simulink library "ModG_Vehiculo"  (R2018a)
settings: Solver=VariableStepAuto  StartTime=0.0  StopTime=10.0  RelTol=1e-3
undefined symbols (not defined in the file): a1, a2, Auto, b1d, b1i, b2d, b2i, b_sus, g, h, Iyy, Izz, Jw, k_sus, L, m, Rg, T1, T2
libraries: $bdroot x12, ModG_Neumatico x10, ModG_Transformaciones x2
settings Model: Creator=Lisandro Cocca  LastModifiedBy=Lisandro Cocca

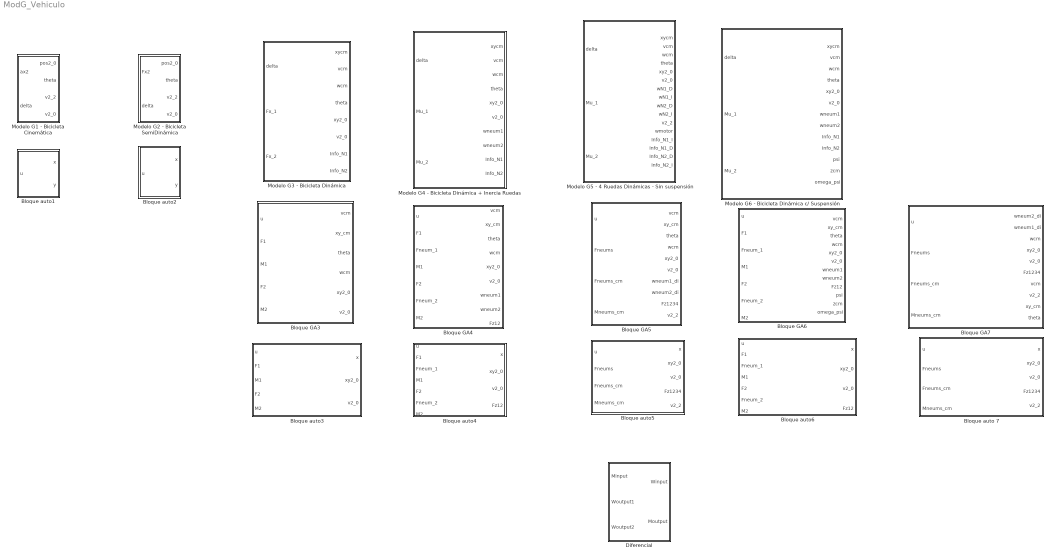
== system ModG_Vehiculo ==
  Bloque GA3 : Subsystem
  Bloque GA4 : Subsystem
  Bloque GA5 : Subsystem
  Bloque GA6 : Subsystem
  Bloque GA7 : Subsystem
  "Bloque auto 7 " : Subsystem
  Bloque auto1 : Subsystem
  Bloque auto2 : Subsystem
  Bloque auto3 : Subsystem
  Bloque auto4 : Subsystem
  Bloque auto5 : Subsystem
  Bloque auto6 : Subsystem
  Diferencial : Subsystem  mask{rel_dif=1}
      mask prompts: rel_dif "Relacion del diferencial 'rel_dif'"
  Modelo G1 - Bicicleta Cinemática : Subsystem  mask{L=L}
      mask prompts: L "Largo del auto "L" [m]"
  Modelo G2 - Bicicleta SemiDinámica : Subsystem  mask{L=L, m=m}
      mask prompts: L "Largo del auto "L" [m]"; m "Masa del auto "m" [kg]"
  Modelo G3 - Bicicleta Dinámica : Subsystem  mask{m=0, Izz=0, L=0, a2=0, a1=0, g=9.81}
      mask prompts: m "Masa del auto 'm' [kg]"; Izz "Momento de inercia respecto eje Z 'Izz' [kg/m^2]"; L "Distancia entre ejes 'L' [m]"; a2 "Distancia CM-Eje trasero 'a2' [m] (Numero positivo)"; a1 "Distancia CM-Eje delantero 'a1' [m] (Numero positivo)"; g "Aceleracion de la gravedad 'g' [m/s^2]"
  Modelo G4 - Bicicleta Dinámica + Inercia Ruedas : Subsystem  mask{m=0, Izz=0, L=0, a2=0, a1=0, h=0, g=9.81, GR=0, Rg=0, Jw=0}
      mask prompts: m "Masa del auto 'm' [kg]"; Izz "Momento de inercia respecto eje Z 'Izz' [kg/m^2]"; L "Distancia entre ejes 'L' [m]"; a2 "Distancia CM-Eje trasero 'a2' [m] (Numero positivo)"; a1 "Distancia CM-Eje delantero 'a1' [m] (Numero positivo)"; h "Altura del centro de masa 'h' [m]"; g "Aceleracion de la gravedad 'g' [m/s^2]"; GR "Gear Ratio 'GR'"; Rg "Radio Neumático 'Rg'"; Jw "Inercia Neumático 'Jw'"
  Modelo G5 - 4 Ruedas Dinámicas - Sin suspensión : Subsystem  mask{m=0, Izz=0, L=0, a2=0, a1=0, T1=0, b1d=0, b1i=0, b2d=0, b2i=0, T2=0, h=0, g=9.81, GR=1, Rg=0, Jw=0}
      mask prompts: m "Masa del auto 'm' [kg]"; Izz "Momento de inercia respecto eje Z 'Izz' [kg/m^2]"; L "Distancia entre ejes 'L' [m]"; a2 "Distancia CM-Eje trasero 'a2' [m] (Numero positivo)"; a1 "Distancia CM-Eje delantero 'a1' [m] (Numero positivo)"; T1 "Trocha delantera 'T1' [m]"; b1d "Distancia lateral del neumatico delatenro derecho al CM 'b1d'"; b1i "Distancia lateral del neumatico delantero izquierdo al CM 'b1i'"; b2d "Distancia lateral del neumatico trasero derecho al CM 'b2d'"; b2i "Distancia lateral del neumatico trasero izquierdo al CM 'b2i'"; T2 "Trocha trasera 'T2' [m]"; h "Altura del centro de masa 'h' [m]"; g "Aceleracion de la gravedad 'g' [m/s^2]"; GR "Gear Ratio 'GR'"; Rg "Radio Neumático 'Rg'"; Jw "Inercia Neumático 'Jw'"
  Modelo G6 - Bicicleta Dinámica c/ Suspensión : Subsystem  mask{m=0, Izz=0, Iyy=0, L=0, a2=0, a1=0, g=0, GR=0, Rg=0, Jw=0, k_sus=0, b_sus=0, h=0}
      mask prompts: m "Masa del auto 'm' [kg]"; Izz "Momento de inercia respecto eje Z 'Izz' [kg*m^2]"; Iyy "Momento de inercia respecto eje Y 'Iyy' [kg/m^2]"; L "Distancia entre ejes 'L' [m}"; a2 "Distancia CM- Eje trasero 'a2' [m] (Numero positivo)"; a1 "Distancia CM- Eje delantero 'a1' [m] (Numero positivo)"; g "Aceleración de la gravedad 'g' [m/s^2]"; GR "Gear Ratio 'GR'"; Rg "Radio Neumatico 'Rg'"; Jw "Inercia Neumático 'Jw'"; k_sus "Resorte suspensión 'k_sus'"; b_sus "Amortiguador suspensión 'b_sus'"; h "Altura del CM 'h'"

== system ModG_Vehiculo/Bloque GA3 ==
  u : Inport
  F1 : Inport  Port=2
  M1 : Inport  Port=3
  F2 : Inport  Port=4
  M2 : Inport  Port=5
  Bloque auto3 : $bdroot/Bloque auto3
  _theta : Selector  IndexOptions=Index vector (dialog)  Indices=[3]  OutputSizes=1
  _vcm : Selector  IndexOptions=Index vector (dialog)  Indices=[4 5]  OutputSizes=1
  _wcm : Selector  IndexOptions=Index vector (dialog)  Indices=[6]  OutputSizes=1
  _xycm : Selector  IndexOptions=Index vector (dialog)  Indices=[1 2]  OutputSizes=1
  vcm : Outport
  "xy_cm " : Outport  Port=2
  theta : Outport  Port=3
  wcm : Outport  Port=4
  xy2_0 : Outport  Port=5
  v2_0 : Outport  Port=6
  wires:
  u/1 -> Bloque auto3/1
  M2/1 -> Bloque auto3/5
  Bloque auto3/2 -> xy2_0/1
  Bloque auto3/1 -> _theta/1, _wcm/1, _vcm/1, _xycm/1
  _xycm/1 -> "xy_cm "/1
  M1/1 -> Bloque auto3/3
  F1/1 -> Bloque auto3/2
  F2/1 -> Bloque auto3/4
  _theta/1 -> theta/1
  Bloque auto3/3 -> v2_0/1
  _wcm/1 -> wcm/1
  _vcm/1 -> vcm/1

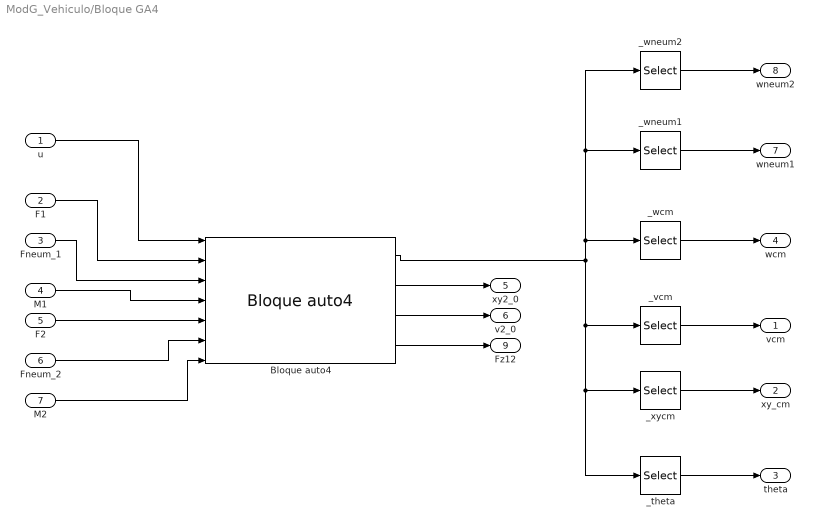
== system ModG_Vehiculo/Bloque GA4 ==
  u : Inport
  F1 : Inport  Port=2
  Fneum_1 : Inport  Port=3
  M1 : Inport  Port=4
  F2 : Inport  Port=5
  Fneum_2 : Inport  Port=6
  M2 : Inport  Port=7
  Bloque auto4 : $bdroot/Bloque auto4
  _theta : Selector  IndexOptions=Index vector (dialog)  Indices=[3]  OutputSizes=1
  _vcm : Selector  IndexOptions=Index vector (dialog)  Indices=[4 5]  OutputSizes=1
  _wcm : Selector  IndexOptions=Index vector (dialog)  Indices=[6]  OutputSizes=1
  _wneum1 : Selector  IndexOptions=Index vector (dialog)  Indices=[7]  OutputSizes=1
  _wneum2 : Selector  IndexOptions=Index vector (dialog)  Indices=[8]  OutputSizes=1
  _xycm : Selector  IndexOptions=Index vector (dialog)  Indices=[1 2]  OutputSizes=1
  vcm : Outport
  "xy_cm " : Outport  Port=2
  theta : Outport  Port=3
  wcm : Outport  Port=4
  xy2_0 : Outport  Port=5
  v2_0 : Outport  Port=6
  wneum1 : Outport  Port=7
  wneum2 : Outport  Port=8
  Fz12 : Outport  Port=9
  wires:
  _xycm/1 -> "xy_cm "/1
  _vcm/1 -> vcm/1
  Bloque auto4/3 -> v2_0/1
  u/1 -> Bloque auto4/1
  _theta/1 -> theta/1
  Bloque auto4/1 -> _theta/1, _xycm/1, _vcm/1, _wneum2/1, _wneum1/1, _wcm/1
  F1/1 -> Bloque auto4/2
  Bloque auto4/2 -> xy2_0/1
  _wcm/1 -> wcm/1
  _wneum2/1 -> wneum2/1
  _wneum1/1 -> wneum1/1
  Fneum_1/1 -> Bloque auto4/3
  M2/1 -> Bloque auto4/7
  F2/1 -> Bloque auto4/5
  Fneum_2/1 -> Bloque auto4/6
  M1/1 -> Bloque auto4/4
  Bloque auto4/4 -> Fz12/1

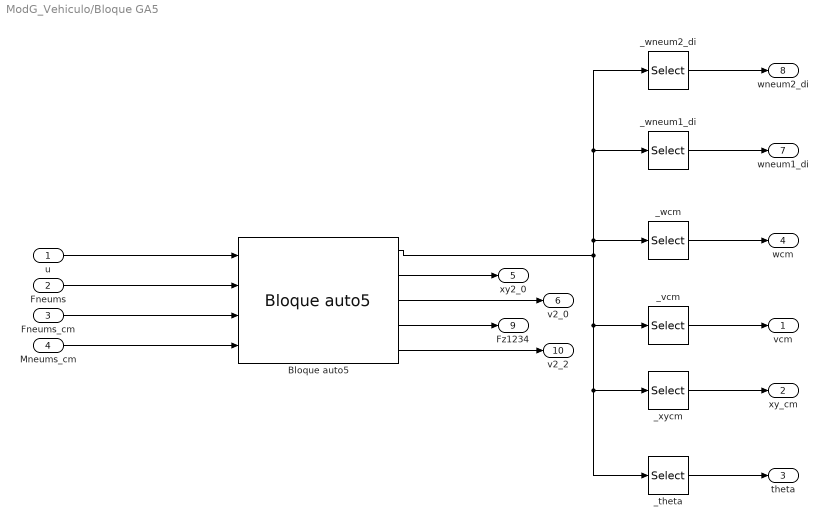
== system ModG_Vehiculo/Bloque GA5 ==
  u : Inport
  Fneums : Inport  Port=2
  Fneums_cm : Inport  Port=3
  Mneums_cm : Inport  Port=4
  Bloque auto5 : $bdroot/Bloque auto5
  _theta : Selector  IndexOptions=Index vector (dialog)  Indices=[3]  OutputSizes=1
  _vcm : Selector  IndexOptions=Index vector (dialog)  Indices=[4 5]  OutputSizes=1
  _wcm : Selector  IndexOptions=Index vector (dialog)  Indices=[6]  OutputSizes=1
  _wneum1_di : Selector  IndexOptions=Index vector (dialog)  Indices=[7 8]  OutputSizes=1
  _wneum2_di : Selector  IndexOptions=Index vector (dialog)  Indices=[9 10]  OutputSizes=1
  _xycm : Selector  IndexOptions=Index vector (dialog)  Indices=[1 2]  OutputSizes=1
  vcm : Outport
  "xy_cm " : Outport  Port=2
  theta : Outport  Port=3
  wcm : Outport  Port=4
  xy2_0 : Outport  Port=5
  v2_0 : Outport  Port=6
  wneum1_di : Outport  Port=7
  wneum2_di : Outport  Port=8
  Fz1234 : Outport  Port=9
  v2_2 : Outport  Port=10
  wires:
  _xycm/1 -> "xy_cm "/1
  _vcm/1 -> vcm/1
  Bloque auto5/3 -> v2_0/1
  u/1 -> Bloque auto5/1
  _theta/1 -> theta/1
  Bloque auto5/1 -> _theta/1, _xycm/1, _vcm/1, _wneum2_di/1, _wneum1_di/1, _wcm/1
  Fneums/1 -> Bloque auto5/2
  Bloque auto5/2 -> xy2_0/1
  _wcm/1 -> wcm/1
  _wneum2_di/1 -> wneum2_di/1
  _wneum1_di/1 -> wneum1_di/1
  Fneums_cm/1 -> Bloque auto5/3
  Mneums_cm/1 -> Bloque auto5/4
  Bloque auto5/4 -> Fz1234/1
  Bloque auto5/5 -> v2_2/1

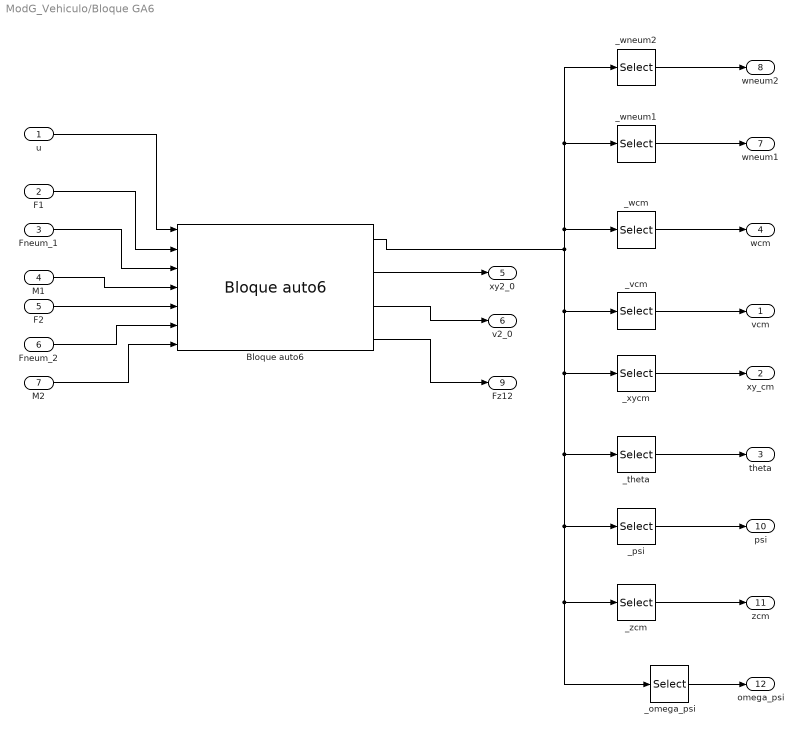
== system ModG_Vehiculo/Bloque GA6 ==
  u : Inport
  F1 : Inport  Port=2
  Fneum_1 : Inport  Port=3
  M1 : Inport  Port=4
  F2 : Inport  Port=5
  Fneum_2 : Inport  Port=6
  M2 : Inport  Port=7
  Bloque auto6 : $bdroot/Bloque auto6
  _omega_psi : Selector  IndexOptions=Index vector (dialog)  Indices=[10]  OutputSizes=1
  _psi : Selector  IndexOptions=Index vector (dialog)  Indices=[9]  OutputSizes=1
  _theta : Selector  IndexOptions=Index vector (dialog)  Indices=[3]  OutputSizes=1
  _vcm : Selector  IndexOptions=Index vector (dialog)  Indices=[4 5]  OutputSizes=1
  _wcm : Selector  IndexOptions=Index vector (dialog)  Indices=[6]  OutputSizes=1
  _wneum1 : Selector  IndexOptions=Index vector (dialog)  Indices=[7]  OutputSizes=1
  _wneum2 : Selector  IndexOptions=Index vector (dialog)  Indices=[8]  OutputSizes=1
  _xycm : Selector  IndexOptions=Index vector (dialog)  Indices=[1 2]  OutputSizes=1
  _zcm : Selector  IndexOptions=Index vector (dialog)  Indices=[11]  OutputSizes=1
  vcm : Outport
  "xy_cm " : Outport  Port=2
  theta : Outport  Port=3
  wcm : Outport  Port=4
  xy2_0 : Outport  Port=5
  v2_0 : Outport  Port=6
  wneum1 : Outport  Port=7
  wneum2 : Outport  Port=8
  Fz12 : Outport  Port=9
  psi : Outport  Port=10
  zcm : Outport  Port=11
  omega_psi : Outport  Port=12
  wires:
  _wneum2/1 -> wneum2/1
  Bloque auto6/3 -> v2_0/1
  M2/1 -> Bloque auto6/7
  _wcm/1 -> wcm/1
  _xycm/1 -> "xy_cm "/1
  Fneum_2/1 -> Bloque auto6/6
  F1/1 -> Bloque auto6/2
  _vcm/1 -> vcm/1
  _wneum1/1 -> wneum1/1
  Bloque auto6/4 -> Fz12/1
  u/1 -> Bloque auto6/1
  Bloque auto6/2 -> xy2_0/1
  F2/1 -> Bloque auto6/5
  _theta/1 -> theta/1
  Fneum_1/1 -> Bloque auto6/3
  M1/1 -> Bloque auto6/4
  _psi/1 -> psi/1
  Bloque auto6/1 -> _omega_psi/1, _zcm/1, _psi/1, _theta/1, _xycm/1, _vcm/1, _wneum2/1, _wneum1/1, _wcm/1
  _zcm/1 -> zcm/1
  _omega_psi/1 -> omega_psi/1

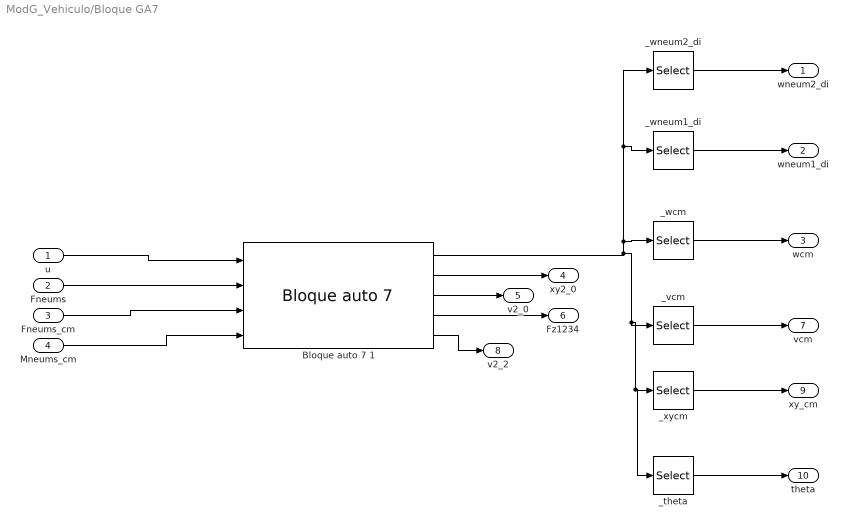
== system ModG_Vehiculo/Bloque GA7 ==
  u : Inport
  Fneums : Inport  Port=2
  Fneums_cm : Inport  Port=3
  Mneums_cm : Inport  Port=4
  Bloque auto 7 1 : $bdroot/Bloque auto 7 
  _theta : Selector  IndexOptions=Index vector (dialog)  Indices=[3]  OutputSizes=1
  _vcm : Selector  IndexOptions=Index vector (dialog)  Indices=[4 5]  OutputSizes=1
  _wcm : Selector  IndexOptions=Index vector (dialog)  Indices=[6]  OutputSizes=1
  _wneum1_di : Selector  IndexOptions=Index vector (dialog)  Indices=[7 8]  OutputSizes=1
  _wneum2_di : Selector  IndexOptions=Index vector (dialog)  Indices=[9 10]  OutputSizes=1
  _xycm : Selector  IndexOptions=Index vector (dialog)  Indices=[1 2]  OutputSizes=1
  wneum2_di : Outport
  wneum1_di : Outport  Port=2
  wcm : Outport  Port=3
  xy2_0 : Outport  Port=4
  v2_0 : Outport  Port=5
  Fz1234 : Outport  Port=6
  vcm : Outport  Port=7
  v2_2 : Outport  Port=8
  "xy_cm " : Outport  Port=9
  theta : Outport  Port=10
  wires:
  _theta/1 -> theta/1
  _vcm/1 -> vcm/1
  Bloque auto 7 1/3 -> v2_0/1
  _wcm/1 -> wcm/1
  _wneum2_di/1 -> wneum2_di/1
  u/1 -> Bloque auto 7 1/1
  _wneum1_di/1 -> wneum1_di/1
  _xycm/1 -> "xy_cm "/1
  Bloque auto 7 1/4 -> Fz1234/1
  Fneums/1 -> Bloque auto 7 1/2
  Fneums_cm/1 -> Bloque auto 7 1/3
  Bloque auto 7 1/1 -> _theta/1, _xycm/1, _vcm/1, _wcm/1, _wneum1_di/1, _wneum2_di/1
  Bloque auto 7 1/2 -> xy2_0/1
  Mneums_cm/1 -> Bloque auto 7 1/4
  Bloque auto 7 1/5 -> v2_2/1

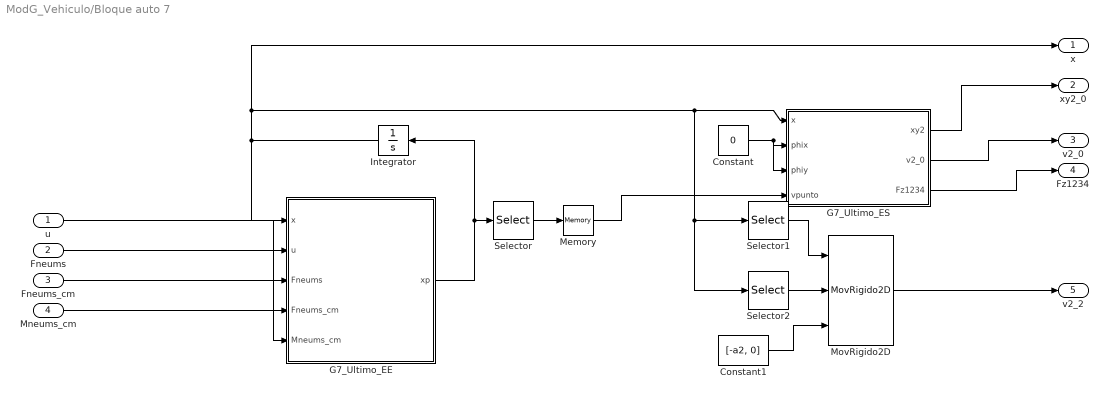
== system ModG_Vehiculo/Bloque auto 7  ==
  u : Inport
  Fneums : Inport  Port=2
  Fneums_cm : Inport  Port=3
  Mneums_cm : Inport  Port=4
  Constant : Constant  Value=0
  Constant1 : Constant  Value=[-a2, 0]
  G7_Ultimo_EE : MATLAB Function  TreatAsAtomicUnit=on
  G7_Ultimo_ES : MATLAB Function  TreatAsAtomicUnit=on
  Integrator : Integrator
  Memory : Memory
  MovRigido2D : ModG_Transformaciones/MovRigido2D
  Selector : Selector  IndexOptions=Index vector (dialog)  Indices=[4, 5]  OutputSizes=1
  Selector1 : Selector  IndexOptions=Index vector (dialog)  Indices=[4 5]  OutputSizes=1
  Selector2 : Selector  IndexOptions=Index vector (dialog)  Indices=6  OutputSizes=1
  x : Outport
  xy2_0 : Outport  Port=2
  v2_0 : Outport  Port=3
  Fz1234 : Outport  Port=4
  v2_2 : Outport  Port=5
  wires:
  G7_Ultimo_EE/1(xp) -> Selector/1, Integrator/1
  Integrator/1 -> G7_Ultimo_EE/1(x), x/1, Selector2/1, Selector1/1, G7_Ultimo_ES/1(x)
  Mneums_cm/1 -> G7_Ultimo_EE/5(Mneums_cm)
  Memory/1 -> G7_Ultimo_ES/4(vpunto)
  G7_Ultimo_ES/1(xy2) -> xy2_0/1
  Fneums/1 -> G7_Ultimo_EE/3(Fneums)
  Selector2/1 -> MovRigido2D/2
  MovRigido2D/1 -> v2_2/1
  G7_Ultimo_ES/3(Fz1234) -> Fz1234/1
  u/1 -> G7_Ultimo_EE/2(u)
  Selector1/1 -> MovRigido2D/1
  Fneums_cm/1 -> G7_Ultimo_EE/4(Fneums_cm)
  Constant/1 -> G7_Ultimo_ES/3(phiy), G7_Ultimo_ES/2(phix)
  Selector/1 -> Memory/1
  Constant1/1 -> MovRigido2D/3
  G7_Ultimo_ES/2(v2_0) -> v2_0/1

== system ModG_Vehiculo/Bloque auto1 ==
  u : Inport
  EE_G1 : MATLAB Function  TreatAsAtomicUnit=on
  ES_G1 : MATLAB Function  TreatAsAtomicUnit=on
  Integrator : Integrator
  x : Outport
  y : Outport  Port=2
  wires:
  Integrator/1 -> x/1, ES_G1/1(x), EE_G1/1(x)
  ES_G1/1(y) -> y/1
  EE_G1/1(xp) -> Integrator/1
  u/1 -> ES_G1/2(u), EE_G1/2(u)

== system ModG_Vehiculo/Bloque auto2 ==
  u : Inport
  EE : MATLAB Function  TreatAsAtomicUnit=on
  ES : MATLAB Function  TreatAsAtomicUnit=on
  Integrator : Integrator
  x : Outport
  y : Outport  Port=2
  wires:
  EE/1(xp) -> Integrator/1
  Integrator/1 -> x/1, ES/1(x), EE/1(x)
  u/1 -> ES/2(u), EE/2(u)
  ES/1(y) -> y/1

== system ModG_Vehiculo/Bloque auto3 ==
  u : Inport
  F1 : Inport  Port=2
  M1 : Inport  Port=3
  F2 : Inport  Port=4
  M2 : Inport  Port=5
  G3_BiciSD_EE : MATLAB Function  TreatAsAtomicUnit=on
  G3_BiciSD_ES : MATLAB Function  TreatAsAtomicUnit=on
  Integrator : Integrator
  x : Outport
  xy2_0 : Outport  Port=2
  v2_0 : Outport  Port=3
  wires:
  F1/1 -> G3_BiciSD_EE/3(F1)
  G3_BiciSD_ES/2(v2_0) -> v2_0/1
  Integrator/1 -> G3_BiciSD_EE/1(x), x/1, G3_BiciSD_ES/1(x)
  G3_BiciSD_ES/1(xy2) -> xy2_0/1
  G3_BiciSD_EE/1(xp) -> Integrator/1
  u/1 -> G3_BiciSD_EE/2(u)
  F2/1 -> G3_BiciSD_EE/4(F2)
  M1/1 -> G3_BiciSD_EE/5(M1)
  M2/1 -> G3_BiciSD_EE/6(M2)

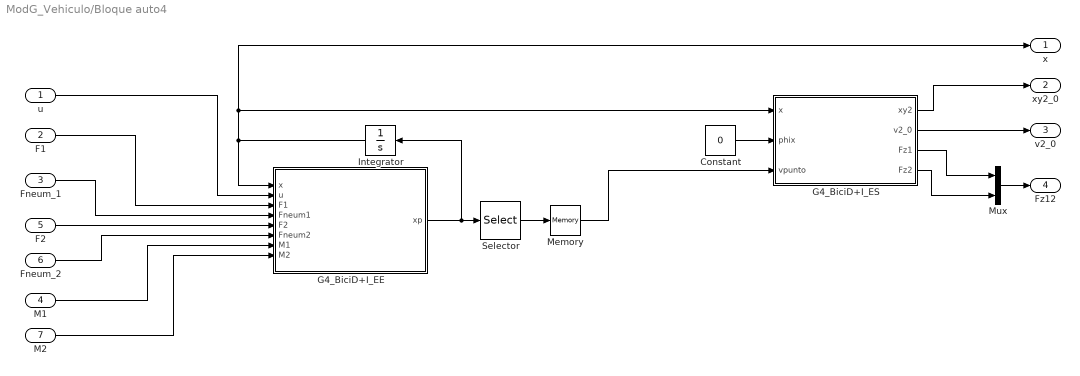
== system ModG_Vehiculo/Bloque auto4 ==
  u : Inport
  F1 : Inport  Port=2
  Fneum_1 : Inport  Port=3
  M1 : Inport  Port=4
  F2 : Inport  Port=5
  Fneum_2 : Inport  Port=6
  M2 : Inport  Port=7
  Constant : Constant  Value=0
  G4_BiciD+I_EE : MATLAB Function  TreatAsAtomicUnit=on
  G4_BiciD+I_ES : MATLAB Function  TreatAsAtomicUnit=on
  Integrator : Integrator
  Memory : Memory
  Mux : Mux  Inputs=2
  Selector : Selector  InputPortWidth=8  IndexOptions=Index vector (dialog)  Indices=4  OutputSizes=1
  x : Outport
  xy2_0 : Outport  Port=2
  v2_0 : Outport  Port=3
  Fz12 : Outport  Port=4
  wires:
  F2/1 -> G4_BiciD+I_EE/5(F2)
  G4_BiciD+I_EE/1(xp) -> Selector/1, Integrator/1
  Integrator/1 -> G4_BiciD+I_EE/1(x), G4_BiciD+I_ES/1(x), x/1
  u/1 -> G4_BiciD+I_EE/2(u)
  G4_BiciD+I_ES/2(v2_0) -> v2_0/1
  M1/1 -> G4_BiciD+I_EE/7(M1)
  G4_BiciD+I_ES/1(xy2) -> xy2_0/1
  F1/1 -> G4_BiciD+I_EE/3(F1)
  M2/1 -> G4_BiciD+I_EE/8(M2)
  Fneum_1/1 -> G4_BiciD+I_EE/4(Fneum1)
  Fneum_2/1 -> G4_BiciD+I_EE/6(Fneum2)
  Selector/1 -> Memory/1
  Memory/1 -> G4_BiciD+I_ES/3(vpunto)
  Mux/1 -> Fz12/1
  G4_BiciD+I_ES/3(Fz1) -> Mux/1
  G4_BiciD+I_ES/4(Fz2) -> Mux/2
  Constant/1 -> G4_BiciD+I_ES/2(phix)

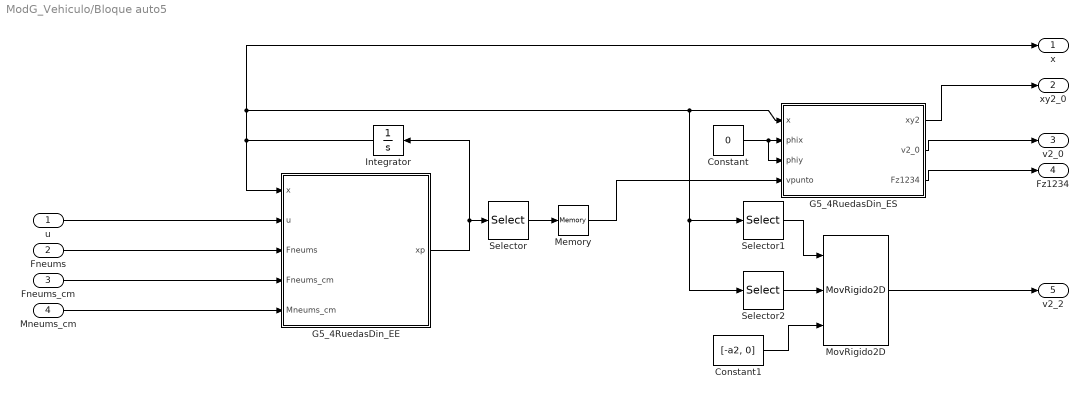
== system ModG_Vehiculo/Bloque auto5 ==
  u : Inport
  Fneums : Inport  Port=2
  Fneums_cm : Inport  Port=3
  Mneums_cm : Inport  Port=4
  Constant : Constant  Value=0
  Constant1 : Constant  Value=[-a2, 0]
  G5_4RuedasDin_EE : MATLAB Function  TreatAsAtomicUnit=on
  G5_4RuedasDin_ES : MATLAB Function  TreatAsAtomicUnit=on
  Integrator : Integrator
  Memory : Memory
  MovRigido2D : ModG_Transformaciones/MovRigido2D
  Selector : Selector  IndexOptions=Index vector (dialog)  Indices=[4, 5]  OutputSizes=1
  Selector1 : Selector  IndexOptions=Index vector (dialog)  Indices=[4 5]  OutputSizes=1
  Selector2 : Selector  IndexOptions=Index vector (dialog)  Indices=6  OutputSizes=1
  x : Outport
  xy2_0 : Outport  Port=2
  v2_0 : Outport  Port=3
  Fz1234 : Outport  Port=4
  v2_2 : Outport  Port=5
  wires:
  Mneums_cm/1 -> G5_4RuedasDin_EE/5(Mneums_cm)
  G5_4RuedasDin_EE/1(xp) -> Selector/1, Integrator/1
  u/1 -> G5_4RuedasDin_EE/2(u)
  G5_4RuedasDin_ES/2(v2_0) -> v2_0/1
  G5_4RuedasDin_ES/1(xy2) -> xy2_0/1
  Fneums/1 -> G5_4RuedasDin_EE/3(Fneums)
  Fneums_cm/1 -> G5_4RuedasDin_EE/4(Fneums_cm)
  Selector/1 -> Memory/1
  Memory/1 -> G5_4RuedasDin_ES/4(vpunto)
  G5_4RuedasDin_ES/3(Fz1234) -> Fz1234/1
  Constant/1 -> G5_4RuedasDin_ES/3(phiy), G5_4RuedasDin_ES/2(phix)
  Selector1/1 -> MovRigido2D/1
  Selector2/1 -> MovRigido2D/2
  Integrator/1 -> G5_4RuedasDin_EE/1(x), Selector2/1, Selector1/1, G5_4RuedasDin_ES/1(x), x/1
  Constant1/1 -> MovRigido2D/3
  MovRigido2D/1 -> v2_2/1

== system ModG_Vehiculo/Bloque auto6 ==
  u : Inport
  F1 : Inport  Port=2
  Fneum_1 : Inport  Port=3
  M1 : Inport  Port=4
  F2 : Inport  Port=5
  Fneum_2 : Inport  Port=6
  M2 : Inport  Port=7
  G6_BiciDI_ES : MATLAB Function  TreatAsAtomicUnit=on
  G6_BiciD_EE : MATLAB Function  TreatAsAtomicUnit=on
  Integrator : Integrator
  Mux : Mux  Inputs=2
  x : Outport
  xy2_0 : Outport  Port=2
  v2_0 : Outport  Port=3
  Fz12 : Outport  Port=4
  wires:
  u/1 -> G6_BiciD_EE/2(u)
  G6_BiciDI_ES/2(v2_0) -> v2_0/1
  Integrator/1 -> G6_BiciD_EE/1(x), x/1, G6_BiciDI_ES/1(x)
  G6_BiciD_EE/1(xp) -> Integrator/1
  Fneum_1/1 -> G6_BiciD_EE/4(Fneum1)
  M2/1 -> G6_BiciD_EE/8(M2)
  Mux/1 -> Fz12/1
  F1/1 -> G6_BiciD_EE/3(F1)
  M1/1 -> G6_BiciD_EE/7(M1)
  Fneum_2/1 -> G6_BiciD_EE/6(Fneum2)
  F2/1 -> G6_BiciD_EE/5(F2)
  G6_BiciDI_ES/1(xy2) -> xy2_0/1
  G6_BiciDI_ES/3(Fz1) -> Mux/1
  G6_BiciDI_ES/4(Fz2) -> Mux/2

== system ModG_Vehiculo/Diferencial ==
  Minput : Inport
  Woutput1 : Inport  Port=2
  Woutput2 : Inport  Port=3
  Gain : Gain  Gain=Auto.GR
  Gain1 : Gain  Gain=1/Auto.GR
  Sum : Sum  Inputs=+|+
  Winput : Outport
  Moutput : Outport  Port=2
  wires:
  Minput/1 -> Gain/1
  Gain/1 -> Moutput/1
  Woutput1/1 -> Sum/1
  Sum/1 -> Gain1/1
  Gain1/1 -> Winput/1
  Woutput2/1 -> Sum/2

== system ModG_Vehiculo/Modelo G1 - Bicicleta Cinemática ==
  note: Bloque GA1
  ax2 : Inport
  delta : Inport  Port=2
  Constant : Constant  Value=0
  Modelo auto1 : $bdroot/Bloque auto1
  Mux : Mux  Inputs=2
  Mux1 : Mux  Inputs=2
  Selector : Selector  IndexOptions=Index vector (dialog)  Indices=[1 2]  OutputSizes=1
  Selector1 : Selector  IndexOptions=Index vector (dialog)  Indices=[3]  OutputSizes=1
  Selector2 : Selector  IndexOptions=Index vector (dialog)  Indices=[4]  OutputSizes=1
  Selector3 : Selector  IndexOptions=Index vector (dialog)  Indices=[1 2]  OutputSizes=1
  pos2_0 : Outport
  theta : Outport  Port=2
  v2_2 : Outport  Port=3
  v2_0 : Outport  Port=4
  wires:
  Selector/1 -> pos2_0/1
  Selector1/1 -> theta/1
  Mux1/1 -> v2_2/1
  Selector3/1 -> v2_0/1
  delta/1 -> Mux/2
  Constant/1 -> Mux1/2
  Modelo auto1/2 -> Selector3/1
  Selector2/1 -> Mux1/1
  Mux/1 -> Modelo auto1/1
  Modelo auto1/1 -> Selector2/1, Selector1/1, Selector/1
  ax2/1 -> Mux/1

== system ModG_Vehiculo/Modelo G2 - Bicicleta SemiDinámica ==
  note: Bloque GA2
  Fx2 : Inport
  delta : Inport  Port=2
  Bloque auto2 : $bdroot/Bloque auto2
  Constant : Constant  Value=0
  Mux : Mux  Inputs=2
  Mux1 : Mux  Inputs=2
  Selector : Selector  IndexOptions=Index vector (dialog)  Indices=[1 2]  OutputSizes=1
  Selector1 : Selector  IndexOptions=Index vector (dialog)  Indices=[3]  OutputSizes=1
  Selector2 : Selector  IndexOptions=Index vector (dialog)  Indices=[4]  OutputSizes=1
  Selector3 : Selector  IndexOptions=Index vector (dialog)  Indices=[1 2]  OutputSizes=1
  pos2_0 : Outport
  theta : Outport  Port=2
  v2_2 : Outport  Port=3
  v2_0 : Outport  Port=4
  wires:
  Selector/1 -> pos2_0/1
  Selector1/1 -> theta/1
  Mux1/1 -> v2_2/1
  Selector3/1 -> v2_0/1
  delta/1 -> Mux/2
  Selector2/1 -> Mux1/1
  Mux/1 -> Bloque auto2/1
  Bloque auto2/2 -> Selector3/1
  Bloque auto2/1 -> Selector/1, Selector1/1, Selector2/1
  Fx2/1 -> Mux/1
  Constant/1 -> Mux1/2

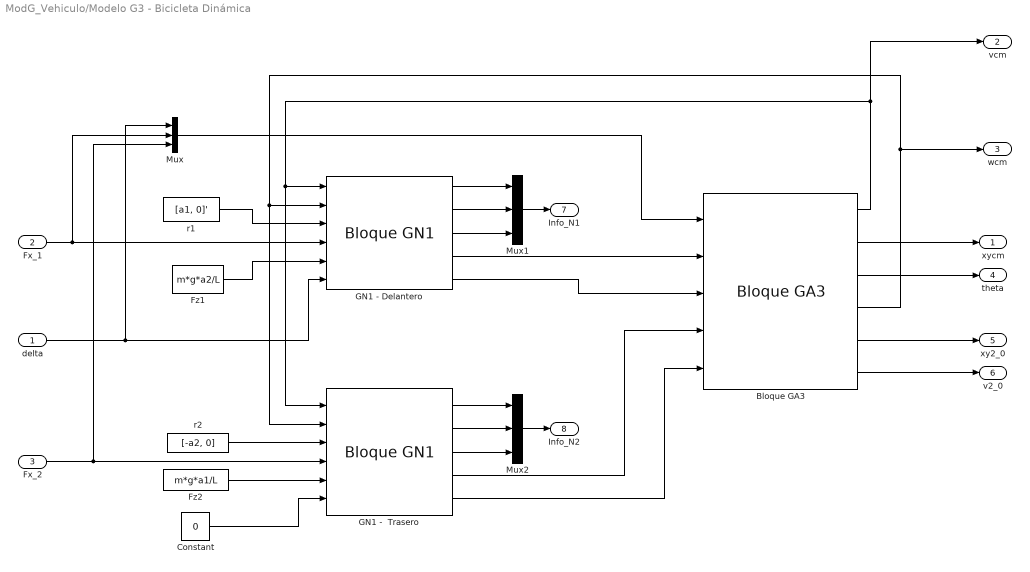
== system ModG_Vehiculo/Modelo G3 - Bicicleta Dinámica ==
  delta : Inport
  Fx_1 : Inport  Port=2
  Fx_2 : Inport  Port=3
  Bloque GA3 : $bdroot/Bloque GA3
  Constant : Constant  Value=0
  Fz1 : Constant  Value=m*g*a2/L
  Fz2 : Constant  Value=m*g*a1/L
  GN1 -  Trasero : ModG_Neumatico/Bloque GN1  mux=1  muy=1  Calfa=5
  GN1 - Delantero : ModG_Neumatico/Bloque GN1  mux=1  muy=1  Calfa=5
  Mux : Mux  Inputs=3
  Mux1 : Mux  Inputs=3
  Mux2 : Mux  Inputs=3
  r1 : Constant  Value=[a1, 0]'  VectorParams1D=off
  r2 : Constant  Value=[-a2, 0]  VectorParams1D=off
  xycm : Outport
  vcm : Outport  Port=2
  wcm : Outport  Port=3
  theta : Outport  Port=4
  xy2_0 : Outport  Port=5
  v2_0 : Outport  Port=6
  Info_N1 : Outport  Port=7
  Info_N2 : Outport  Port=8
  wires:
  delta/1 -> Mux/1, GN1 - Delantero/6
  Fx_2/1 -> Mux/3, GN1 -  Trasero/4
  Fz1/1 -> GN1 - Delantero/5
  r1/1 -> GN1 - Delantero/3
  r2/1 -> GN1 -  Trasero/3
  GN1 - Delantero/1 -> Mux1/1
  Fz2/1 -> GN1 -  Trasero/5
  Constant/1 -> GN1 -  Trasero/6
  GN1 - Delantero/3 -> Mux1/3
  Mux/1 -> Bloque GA3/1
  GN1 - Delantero/4 -> Bloque GA3/2
  GN1 - Delantero/5 -> Bloque GA3/3
  GN1 -  Trasero/4 -> Bloque GA3/4
  Bloque GA3/1 -> GN1 -  Trasero/1, GN1 - Delantero/1, vcm/1
  Bloque GA3/4 -> GN1 -  Trasero/2, GN1 - Delantero/2, wcm/1
  Bloque GA3/2 -> xycm/1
  Bloque GA3/3 -> theta/1
  Bloque GA3/5 -> xy2_0/1
  Bloque GA3/6 -> v2_0/1
  GN1 -  Trasero/5 -> Bloque GA3/5
  Fx_1/1 -> Mux/2, GN1 - Delantero/4
  GN1 - Delantero/2 -> Mux1/2
  Mux1/1 -> Info_N1/1
  Mux2/1 -> Info_N2/1
  GN1 -  Trasero/1 -> Mux2/1
  GN1 -  Trasero/2 -> Mux2/2
  GN1 -  Trasero/3 -> Mux2/3

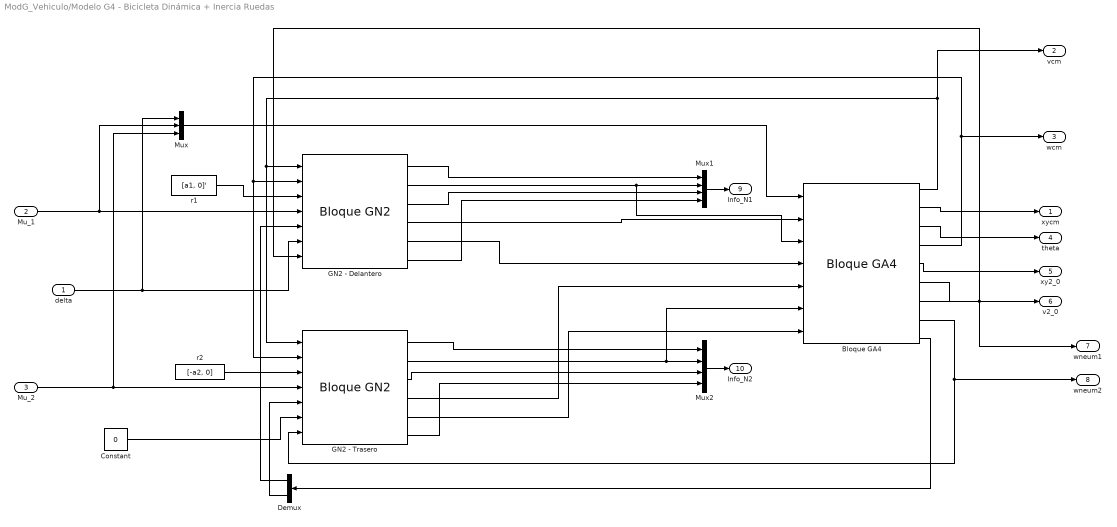
== system ModG_Vehiculo/Modelo G4 - Bicicleta Dinámica + Inercia Ruedas ==
  delta : Inport
  Mu_1 : Inport  Port=2
  Mu_2 : Inport  Port=3
  Bloque GA4 : $bdroot/Bloque GA4
  Constant : Constant  Value=0
  Demux : Demux  Outputs=2
  GN2 - Delantero : ModG_Neumatico/Bloque GN2  muy=Neum.muy  Calfa=Neum.Calfa  low_v=Neum.low_v  mu_s=Neum.mu_s  sc=Neum.sc
  GN2 - Trasero : ModG_Neumatico/Bloque GN2  muy=Neum.muy  Calfa=Neum.Calfa  low_v=Neum.low_v  mu_s=Neum.mu_s  sc=Neum.sc
  Mux : Mux  Inputs=3
  Mux1 : Mux
  Mux2 : Mux
  r1 : Constant  Value=[a1, 0]'  VectorParams1D=off
  r2 : Constant  Value=[-a2, 0]  VectorParams1D=off
  xycm : Outport
  vcm : Outport  Port=2
  wcm : Outport  Port=3
  theta : Outport  Port=4
  xy2_0 : Outport  Port=5
  v2_0 : Outport  Port=6
  wneum1 : Outport  Port=7
  wneum2 : Outport  Port=8
  Info_N1 : Outport  Port=9
  Info_N2 : Outport  Port=10
  wires:
  Mu_1/1 -> GN2 - Delantero/4, Mux/2
  Bloque GA4/2 -> xycm/1
  Bloque GA4/7 -> wneum1/1, GN2 - Delantero/7
  Bloque GA4/6 -> v2_0/1
  Bloque GA4/4 -> wcm/1, GN2 - Trasero/2, GN2 - Delantero/2
  GN2 - Delantero/1 -> Mux1/1
  GN2 - Delantero/3 -> Mux1/3
  delta/1 -> GN2 - Delantero/6, Mux/1
  Bloque GA4/1 -> vcm/1, GN2 - Trasero/1, GN2 - Delantero/1
  r2/1 -> GN2 - Trasero/3
  Constant/1 -> GN2 - Trasero/6
  Mu_2/1 -> Mux/3, GN2 - Trasero/4
  Mux/1 -> Bloque GA4/1
  Bloque GA4/8 -> wneum2/1, GN2 - Trasero/7
  Bloque GA4/3 -> theta/1
  Bloque GA4/5 -> xy2_0/1
  r1/1 -> GN2 - Delantero/3
  GN2 - Trasero/5 -> Bloque GA4/7
  GN2 - Delantero/4 -> Bloque GA4/2
  GN2 - Delantero/5 -> Bloque GA4/4
  GN2 - Trasero/4 -> Bloque GA4/5
  Bloque GA4/9 -> Demux/1
  Demux/1 -> GN2 - Delantero/5
  Demux/2 -> GN2 - Trasero/5
  GN2 - Delantero/2 -> Bloque GA4/3, Mux1/2
  Mux1/1 -> Info_N1/1
  GN2 - Delantero/6 -> Mux1/4
  GN2 - Trasero/3 -> Mux2/3
  GN2 - Trasero/1 -> Mux2/1
  GN2 - Trasero/6 -> Mux2/4
  Mux2/1 -> Info_N2/1
  GN2 - Trasero/2 -> Bloque GA4/6, Mux2/2

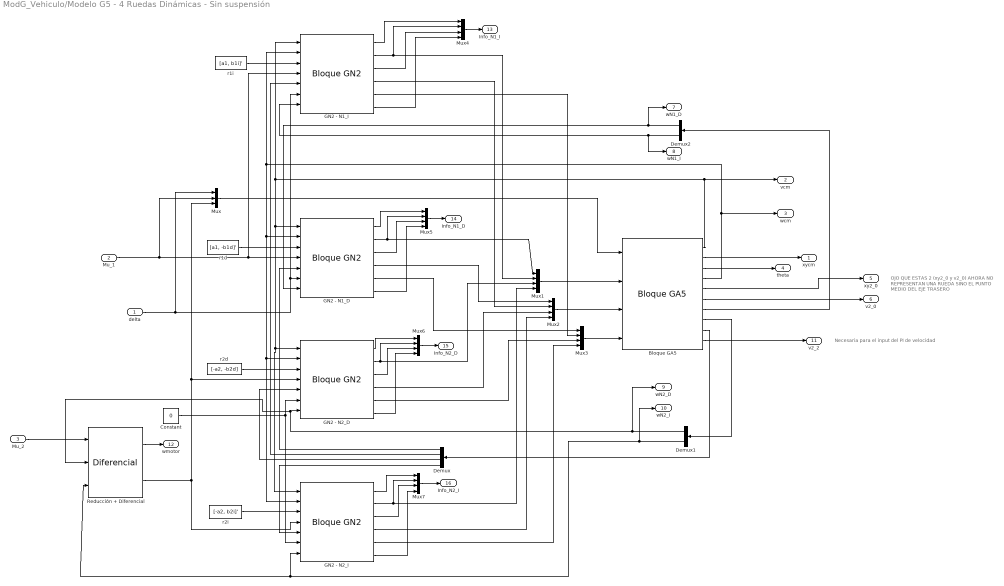
== system ModG_Vehiculo/Modelo G5 - 4 Ruedas Dinámicas - Sin suspensión ==
  note: OJO QUE ESTAS 2 (xy2_0 y v2_0) AHORA NO REPRESENTAN UNA RUEDA
      |  SINO EL PUNTO MEDIO DEL EJE TRASERO
  note: Necesaria para el input del PI de velocidad
  delta : Inport
  Mu_1 : Inport  Port=2
  Mu_2 : Inport  Port=3
  Bloque GA5 : $bdroot/Bloque GA5
  Constant : Constant  Value=0
  Demux : Demux
  Demux1 : Demux  Outputs=2
  Demux2 : Demux  Outputs=2
  GN2 - N1_D : ModG_Neumatico/Bloque GN2  muy=Neum.muy  Calfa=Neum.Calfa  low_v=Neum.low_v  mu_s=Neum.mu_s  sc=Neum.sc
  GN2 - N1_I : ModG_Neumatico/Bloque GN2  muy=Neum.muy  Calfa=Neum.Calfa  low_v=Neum.low_v  mu_s=Neum.mu_s  sc=Neum.sc
  GN2 - N2_D : ModG_Neumatico/Bloque GN2  muy=Neum.muy  Calfa=Neum.Calfa  low_v=Neum.low_v  mu_s=Neum.mu_s  sc=Neum.sc
  GN2 - N2_I : ModG_Neumatico/Bloque GN2  muy=Neum.muy  Calfa=Neum.Calfa  low_v=Neum.low_v  mu_s=Neum.mu_s  sc=Neum.sc
  Mux : Mux  Inputs=3
  Mux{1..7} (7 alike) : Mux
  Reducción + Diferencial : $bdroot/Diferencial  rel_dif=GR
      link override Gain1: Gain=1/Auto.GR
  r1d : Constant  Value=[a1, -b1d]'  VectorParams1D=off
  r1i : Constant  Value=[a1, b1i]'  VectorParams1D=off
  r2d : Constant  Value=[-a2, -b2d]  VectorParams1D=off
  r2i : Constant  Value=[-a2, b2i]'  VectorParams1D=off
  xycm : Outport
  vcm : Outport  Port=2
  wcm : Outport  Port=3
  theta : Outport  Port=4
  xy2_0 : Outport  Port=5
  v2_0 : Outport  Port=6
  wN1_D : Outport  Port=7
  wN1_I : Outport  Port=8
  wN2_D : Outport  Port=9
  wN2_I : Outport  Port=10
  v2_2 : Outport  Port=11
  wmotor : Outport  Port=12
  Info_N1_I : Outport  Port=13
  Info_N1_D : Outport  Port=14
  Info_N2_D : Outport  Port=15
  Info_N2_I : Outport  Port=16
  wires:
  Mu_1/1 -> GN2 - N1_I/4, GN2 - N1_D/4, Mux/2
  Bloque GA5/2 -> xycm/1
  Bloque GA5/7 -> Demux2/1
  Bloque GA5/6 -> v2_0/1
  Bloque GA5/4 -> GN2 - N1_I/2, GN2 - N2_I/2, GN2 - N2_D/2, GN2 - N1_D/2, wcm/1
  delta/1 -> GN2 - N1_D/6, GN2 - N1_I/6, Mux/1
  Bloque GA5/1 -> GN2 - N1_I/1, GN2 - N2_I/1, GN2 - N2_D/1, GN2 - N1_D/1, vcm/1
  r2d/1 -> GN2 - N2_D/3
  GN2 - N2_D/2 -> Mux6/2, Mux1/3
  Constant/1 -> GN2 - N2_I/6, GN2 - N2_D/6
  Mu_2/1 -> Reducción + Diferencial/1
  Mux/1 -> Bloque GA5/1
  Bloque GA5/8 -> Demux1/1
  GN2 - N2_D/6 -> Mux6/4
  GN2 - N1_D/2 -> Mux5/2, Mux1/1
  Bloque GA5/3 -> theta/1
  Bloque GA5/5 -> xy2_0/1
  r1d/1 -> GN2 - N1_D/3
  Bloque GA5/9 -> Demux/1
  Mux1/1 -> Bloque GA5/2
  GN2 - N1_I/2 -> Mux4/2, Mux1/2
  Mux2/1 -> Bloque GA5/3
  GN2 - N1_D/4 -> Mux2/1
  GN2 - N1_I/4 -> Mux2/2
  GN2 - N2_D/4 -> Mux2/3
  GN2 - N2_I/4 -> Mux2/4
  Mux3/1 -> Bloque GA5/4
  GN2 - N1_D/5 -> Mux3/1
  GN2 - N2_D/5 -> Mux3/3
  GN2 - N1_I/5 -> Mux3/2
  GN2 - N2_I/5 -> Mux3/4
  r1i/1 -> GN2 - N1_I/3
  r2i/1 -> GN2 - N2_I/3
  Demux1/1 -> wN2_D/1, Reducción + Diferencial/2, GN2 - N2_D/7
  Demux1/2 -> wN2_I/1, Reducción + Diferencial/3, GN2 - N2_I/7
  Demux2/1 -> wN1_D/1, GN2 - N1_D/7
  Demux2/2 -> wN1_I/1, GN2 - N1_I/7
  GN2 - N1_I/1 -> Mux4/1
  GN2 - N1_I/6 -> Mux4/4
  Bloque GA5/10 -> v2_2/1
  Demux/1 -> GN2 - N1_D/5
  Demux/2 -> GN2 - N1_I/5
  Demux/3 -> GN2 - N2_D/5
  Demux/4 -> GN2 - N2_I/5
  Reducción + Diferencial/2 -> GN2 - N2_I/4, GN2 - N2_D/4, Mux/3
  Reducción + Diferencial/1 -> wmotor/1
  GN2 - N1_I/3 -> Mux4/3
  Mux4/1 -> Info_N1_I/1
  Mux5/1 -> Info_N1_D/1
  GN2 - N1_D/1 -> Mux5/1
  GN2 - N1_D/3 -> Mux5/3
  GN2 - N1_D/6 -> Mux5/4
  Mux6/1 -> Info_N2_D/1
  GN2 - N2_D/1 -> Mux6/1
  GN2 - N2_D/3 -> Mux6/3
  GN2 - N2_I/2 -> Mux1/4, Mux7/2
  Mux7/1 -> Info_N2_I/1
  GN2 - N2_I/6 -> Mux7/4
  GN2 - N2_I/1 -> Mux7/1
  GN2 - N2_I/3 -> Mux7/3

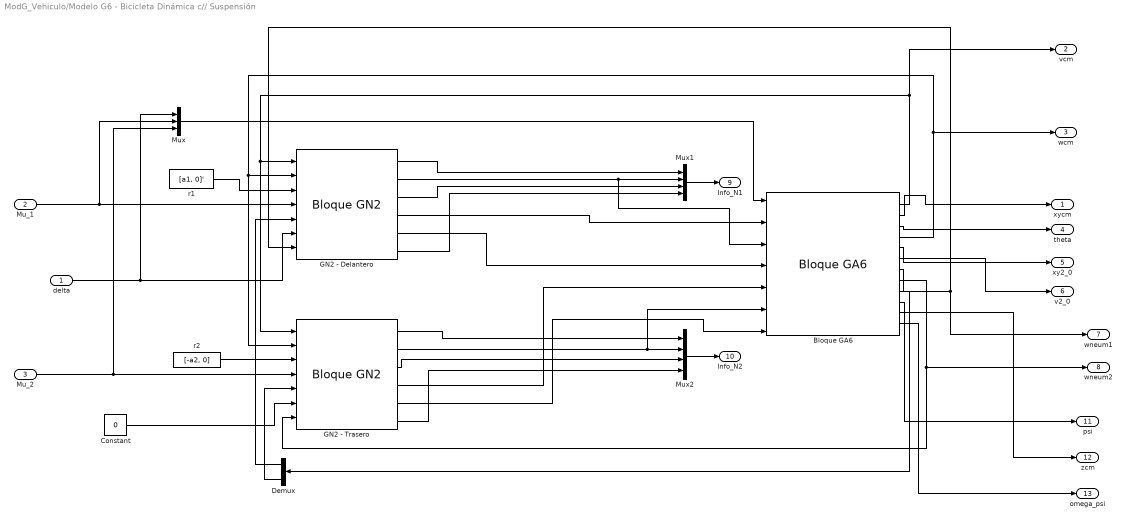
== system ModG_Vehiculo/Modelo G6 - Bicicleta Dinámica c// Suspensión ==
  delta : Inport
  Mu_1 : Inport  Port=2
  Mu_2 : Inport  Port=3
  Bloque GA6 : $bdroot/Bloque GA6
  Constant : Constant  Value=0
  Demux : Demux  Outputs=2
  GN2 - Delantero : ModG_Neumatico/Bloque GN2  muy=Neum.muy  Calfa=Neum.Calfa  low_v=Neum.low_v  mu_s=Neum.mu_s  sc=Neum.sc
  GN2 - Trasero : ModG_Neumatico/Bloque GN2  muy=Neum.muy  Calfa=Neum.Calfa  low_v=Neum.low_v  mu_s=Neum.mu_s  sc=Neum.sc
  Mux : Mux  Inputs=3
  Mux1 : Mux
  Mux2 : Mux
  r1 : Constant  Value=[a1, 0]'  VectorParams1D=off
  r2 : Constant  Value=[-a2, 0]  VectorParams1D=off
  xycm : Outport
  vcm : Outport  Port=2
  wcm : Outport  Port=3
  theta : Outport  Port=4
  xy2_0 : Outport  Port=5
  v2_0 : Outport  Port=6
  wneum1 : Outport  Port=7
  wneum2 : Outport  Port=8
  Info_N1 : Outport  Port=9
  Info_N2 : Outport  Port=10
  psi : Outport  Port=11
  zcm : Outport  Port=12
  omega_psi : Outport  Port=13
  wires:
  Demux/1 -> GN2 - Delantero/5
  Bloque GA6/7 -> wneum1/1, GN2 - Delantero/7
  Mux2/1 -> Info_N2/1
  GN2 - Trasero/2 -> Bloque GA6/6, Mux2/2
  Mux1/1 -> Info_N1/1
  Bloque GA6/4 -> wcm/1, GN2 - Trasero/2, GN2 - Delantero/2
  r1/1 -> GN2 - Delantero/3
  GN2 - Delantero/4 -> Bloque GA6/2
  Demux/2 -> GN2 - Trasero/5
  GN2 - Delantero/3 -> Mux1/3
  Mu_2/1 -> Mux/3, GN2 - Trasero/4
  GN2 - Trasero/3 -> Mux2/3
  Mu_1/1 -> GN2 - Delantero/4, Mux/2
  GN2 - Trasero/5 -> Bloque GA6/7
  Bloque GA6/5 -> xy2_0/1
  Constant/1 -> GN2 - Trasero/6
  GN2 - Trasero/4 -> Bloque GA6/5
  Bloque GA6/3 -> theta/1
  GN2 - Delantero/6 -> Mux1/4
  Bloque GA6/1 -> vcm/1, GN2 - Trasero/1, GN2 - Delantero/1
  GN2 - Delantero/2 -> Bloque GA6/3, Mux1/2
  Bloque GA6/6 -> v2_0/1
  Bloque GA6/8 -> wneum2/1, GN2 - Trasero/7
  GN2 - Delantero/5 -> Bloque GA6/4
  delta/1 -> GN2 - Delantero/6, Mux/1
  r2/1 -> GN2 - Trasero/3
  Bloque GA6/2 -> xycm/1
  Mux/1 -> Bloque GA6/1
  GN2 - Delantero/1 -> Mux1/1
  GN2 - Trasero/1 -> Mux2/1
  GN2 - Trasero/6 -> Mux2/4
  Bloque GA6/9 -> Demux/1
  Bloque GA6/10 -> psi/1
  Bloque GA6/11 -> zcm/1
  Bloque GA6/12 -> omega_psi/1

== matlab function ModG_Vehiculo/Bloque auto4/G4_BiciD+I_EE ==
  data m settings: description=Masa del auto
  data Izz settings: description=Momento de inercia en el eje z respecto al cm
  data: x input; u input; xp output size=8; F1 input; Fneum1 input; F2 input; Fneum2 input; M1 input; M2 input; m parameter; Izz parameter; Jw parameter; Rg parameter
function xp  = G4_BiciDI_EE(x, u, F1, Fneum1, F2, Fneum2, M1, M2, m, Izz, Jw, Rg)
% Modelo semi dinamico (o dinamico simple, ruedas con inercia)
% x: variables de estado [xcm_0, ycm_0, thetacm, vxcm, vycm, omegacm, wneum_1, wneum_2]'
% u: entradas [delta, Mu_1, Mu_2] --> delta es el angulo de direccion y
% Mu_1 Mu_2 son las torques de entrada sobre los neumaticos provistas
% por el motor/frenos
% F1(x,u) y F2(x,u): Fuerzas en los neumaticos delanteros y traseros. Son calculadas
% internamente al sistema por eso no van como entradas
% M1(x,u) y M2(x,u): Momentos sobre el CM producidos por los neumaticos
% xp: dx/dt = Ax + Bu + F(x,u)

A = [   0   0   0   cos(x(3))   -sin(x(3))  0   0   0
        0   0   0   sin(x(3))   cos(x(3))   0   0   0;
        0   0   0   0           0           1   0   0;
        0   0   0   0          0           0   0   0;
        0   0   0   0           0           0   0   0;
        0   0   0   0           0           0   0   0;
        0   0   0   0           0           0   0   0;
        0   0   0   0           0           0   0   0];

B = [   0   0   0;
        0   0   0;
        0   0   0;
        0   0   0;
        0   0   0;
        0   0   0;
        0   1/Jw 0;
        0   0   1/Jw;
    ];

% Las fuerzas y momentos de los neumáticos los trabajo vectorialmente asi
% es mas facil agregar varias ruedas despues.
% Despues voy a pensar de hacer de esto algo como el 'calcVelOffset' porque
% la cuenta es la analoga.
Fres = F1 + F2; % Fuerza total. Se puede parametrizar fácil para varios neumaticos
Mres = M1 + M2; % Vector momento = suma de productos vectoriales

F = [   0;
    0;
    0;
    Fres(1)/m;
    Fres(2)/m;
    Mres(1)/Izz;
    -Fneum1(1)*Rg/Jw;
    -Fneum2(1)*Rg/Jw];

xp = A*x + B*u + F;

== matlab function ModG_Vehiculo/Bloque auto4/G4_BiciD+I_ES ==
  data: x input; phix input; vpunto input; xy2 output size=2; v2_0 output size=2; a2 parameter size=1; Fz1 output; Fz2 output; a1 parameter; m parameter; g parameter; h parameter; L parameter
function [xy2, v2_0, Fz1, Fz2]  = G4_BiciDI_ES(x, phix, vpunto, a2, a1, m, g, h, L)
xy2 = [x(1) - a2*cos(x(3)); x(2) - a2*sin(x(3))];
v2_0 = [cos(x(3)) -sin(x(3)); sin(x(3)) cos(x(3))]*x(4:5);
Fz1 = m*g*(a2/L * cos(phix) - h/L * sin(phix)) - m*vpunto(1)*h/L;
Fz2 = m*g*(a1/L * cos(phix) + h/L * sin(phix)) + m*vpunto(1)*h/L;

== matlab function ModG_Vehiculo/Bloque auto5/G5_4RuedasDin_EE ==
  data m settings: description=Masa del auto
  data Izz settings: description=Momento de inercia en el eje z respecto al cm
  data: x input; u input; xp output size=10; Fneums input; Fneums_cm input; Mneums_cm input; m parameter; Izz parameter; Jw parameter; Rg parameter
function xp  = G5_4RuedasDin_EE(x, u, Fneums, Fneums_cm, Mneums_cm, m, Izz, Jw, Rg)
% Modelo 4 ruedas dinamicas
% x: variables de estado
%[xcm_0, ycm_0, thetacm, vxcm, vycm, omegacm, wneum_1d, wneum_1i, wneum_2d, wneum_2i]'
%[  1      2       3      4     5       6       7           8       9           10]
% u: entradas [delta, Mu_1, Mu_2] --> delta es el angulo de direccion y
% Mu_1 Mu_2 son las torques de entrada sobre los ejes delanteros y traseros
% provistas por el motor
% Fneums: Fuerzas en los neumaticos vistas en su propio sistema
% Fneums_cm: Fuerzas en los neumaticos vistas del sistema CM
% Mneums_cm: Momentos producidos por los neumáticos sobre el CM
% xp: dx/dt = Ax + Bu + F(x,u)

A = [   0   0   0   cos(x(3))   -sin(x(3))  0   0   0   0   0
        0   0   0   sin(x(3))   cos(x(3))   0   0   0   0   0;
        0   0   0   0           0           1   0   0   0   0;
        0   0   0   0          0           0   0   0    0   0;
        0   0   0   0           0           0   0   0   0   0;
        0   0   0   0           0           0   0   0   0   0;
        0   0   0   0           0           0   0   0   0   0;
        0   0   0   0           0           0   0   0   0   0;
        0   0   0   0           0           0   0   0   0   0;
        0   0   0   0           0           0   0   0   0   0];

B = [   0   0   0;
        0   0   0;
        0   0   0;
        0   0   0;
        0   0   0;
        0   0   0;
        0   1/Jw 0;
        0   1/Jw 0;
        0   0   1/Jw;
        0   0   1/Jw;
    ];

% Las fuerzas de neumaticos vienen en matrices de 3xn donde cada columna
% representa el vector fuerza (o momento o velocidad cuando corresponda)
% del neumatico. El orden de estos vectores de la forma:
% Fneums = [F1d, F1i, F2d, F2i] = [Del-Der, Del-Izq, Tra-Der, Tra-Izq]
Fneums = reshape(Fneums, 3,4);
Fneums_cm = reshape(Fneums_cm, 2,4);
%Mneums_cm = reshape(Mneums_cm, 3,4);
Fres = sum(Fneums_cm'); % Fuerza total sobre el CM producida por los neumaticos
Mres = sum(Mneums_cm'); % Momento total sobre el CM producido por los neumaticos

F = [   0;
    0;
    0;
    Fres(1)/m;
    Fres(2)/m;
    Mres(1)/Izz;
    -Fneums(1,1)*Rg/Jw;
    -Fneums(1,2)*Rg/Jw;
    -Fneums(1,3)*Rg/Jw;
    -Fneums(1,4)*Rg/Jw];

xp = A*x + B*u + F;

== matlab function ModG_Vehiculo/Bloque auto2/EE ==
  data: x input size=4; u input size=2; xp output size=4; L parameter size=1; m parameter
function xp = G2_Bicicleta_EE(x,u, L, m)
% Ecuaciones de estado del cinemático puro de bicicleta
% x: vector de variables de estado [x2 y2 theta vx2]'
% u: vector de entradas            [ax2 delta]'
% xp: dx/dt = A(x,u)x + B(x)u
    A = [0  0   0   cos(x(3));
         0  0   0   sin(x(3));
         0  0   0   tan(u(2))/L;
         0  0   0   0];
     
    B = [0  0;
         0  0;
         0  0;
         1/m  0];
     
    xp = A*x + B*u;

== matlab function ModG_Vehiculo/Bloque auto2/ES ==
  data: x input size=4; y output; u input size=2
function y = G2_Bicicleta_ES(x, u)
% Ecuaciones de salida del cinemático puro de bicicleta
% y = Cx + Du
% y = [ v2x_0
%       v2y_0];
    C = [0  0   0   cos(x(3));      % v2x_0
         0  0   0   sin(x(3));];    % v2y_0
    D = [0  0;
         0  0;];

    y = C*x + D*u;

== matlab function ModG_Vehiculo/Bloque auto3/G3_BiciSD_EE ==
  data m settings: description=Masa del auto
  data Izz settings: description=Momento de inercia en el eje z respecto al cm
  data a1 settings: description=Distancia al eje delantero desde el cm (Despues los voy a hacer vectores 2d para agregar facilmente mas ruedas)
  data a2 settings: description=Distancia al eje trasero desde el cm (Despues los voy a hacer vectores 2d para agregar facilmente mas ruedas)
  data: x input; u input; xp output size=6; F1 input; F2 input; M1 input; M2 input; m parameter; Izz parameter; a1 parameter; a2 parameter
function xp  = G3_BiciSD_EE(x, u, F1, F2, M1, M2, m, Izz, a1, a2)
% Modelo semi dinamico (o dinamico simple, ruedas sin inercia)
% x: variables de estado [xcm_0, ycm_0, thetacm, vxcm, vycm, omegacm]'
% u: entradas [delta, Fx_u1, Fx_u2] --> delta es el angulo de direccion y
% Fx_u1 Fx_u2 son las fuerzas longitudinales sobre los neumaticos provistas
% por el motor/frenos
% F1(x,u) y F2(x,u): Fuerzas en los neumaticos delanteros y traseros. Son calculadas
% internamente al sistema por eso no van como entradas
% M1(x,u) y M2(x,u): Momentos sobre el CM producidos por los neumaticos
% xp: dx/dt = Ax + Bu + F(x,u)

A = [   0   0   0   cos(x(3))   -sin(x(3))  0;
        0   0   0   sin(x(3))   cos(x(3))   0;
        0   0   0   0           0           1;
        0   0   0   0           0           0;
        0   0   0   0           0           0;
        0   0   0   0           0           0];

B = [   0   0   0;
        0   0   0;
        0   0   0;
        0   0   0;
        0   0   0;
        0   0   0;];
        
% Las fuerzas y momentos de los neumáticos los trabajo vectorialmente asi
% es mas facil agregar varias ruedas despues.
% Despues voy a pensar de hacer de esto algo como el 'calcVelOffset' porque
% la cuenta es la analoga.
Fneums = F1 + F2; % Fuerza total. Se puede parametrizar fácil para varios neumaticos
Mneums = M1 + M2; % Vector momento = suma de productos vectoriales

F = [   0;
        0;
        0;
        Fneums(1)/m;
        Fneums(2)/m;
        Mneums(1)/Izz;];
    
xp = A*x + B*u + F;

== matlab function ModG_Vehiculo/Bloque auto3/G3_BiciSD_ES ==
  data: x input; xy2 output size=2; v2_0 output size=2; a2 parameter size=1
function [xy2, v2_0]  = G3_BiciSD_ES(x, a2)
xy2 = [x(1) - a2*cos(x(3)); x(2) - a2*sin(x(3))];
v2_0 = [cos(x(3)) -sin(x(3)); sin(x(3)) cos(x(3))]*x(4:5);

== matlab function ModG_Vehiculo/Bloque auto5/G5_4RuedasDin_ES ==
  data: x input; phix input; phiy input; vpunto input; xy2 output size=2; v2_0 output size=2; a2 parameter size=1; Fz1234 output; a1 parameter; m parameter; g parameter; h parameter; L parameter; b1d parameter; b1i parameter; b2d parameter; b2i parameter; T1 parameter; T2 parameter
function [xy2, v2_0, Fz1234]  = G5_4RuedasDin_ES(x, phix, phiy, vpunto, a2, a1, m, g, h, L, b1d, b1i, b2d, b2i, T1, T2)
xy2 = [x(1) - a2*cos(x(3)); x(2) - a2*sin(x(3))];
v2_0 = [cos(x(3)) -sin(x(3)); sin(x(3)) cos(x(3))]*x(4:5);
%Fz1 = m*g*(a2/L * cos(phix) - h/L * sin(phix)); % Estas 2 lineas son sin termino de aceleracion para evitar lazo algebraico
%Fz2 = m*g*(a1/L * cos(phix) + h/L * sin(phix)); % Estas 2 lineas son sin termino de aceleracion para evitar lazo algebraico
%El modelo del auto no es 3d, si no que son 3 submodelos 2d. 1 modelo
%longitudinal y 2 modelos laterales en cada eje. Entonces primero se
%calcula la fuerza normal sobre el eje delantero y trasero con el modelo
%longitudinal y luego esa Fz representa el peso del auto para el calculo de
%transferencia de peso lateral
Fz1 = m*g*(a2/L * cos(phix) - h/L * sin(phix)) - m*vpunto(1)*h/L;
Fz2 = m*g*(a1/L * cos(phix) + h/L * sin(phix)) + m*vpunto(1)*h/L;
Fz1d = Fz1*(b1i/T1 * cos(phiy) + h/T1 * sin(phiy)) + Fz1/g*vpunto(2)*h/T1;
Fz1i = Fz1*(b1d/T1 * cos(phiy) - h/T1 * sin(phiy)) - Fz1/g*vpunto(2)*h/T1;
Fz2d = Fz2*(b2i/T2 * cos(phiy) + h/T2 * sin(phiy)) + Fz2/g*vpunto(2)*h/T2;
Fz2i = Fz2*(b2d/T2 * cos(phiy) - h/T2 * sin(phiy)) - Fz2/g*vpunto(2)*h/T2;
Fz1234 = [Fz1d, Fz1i, Fz2d, Fz2i]';

== matlab function ModG_Vehiculo/Bloque auto6/G6_BiciD_EE ==
  data m settings: description=Masa del auto
  data Izz settings: description=Momento de inercia en el eje z respecto al cm
  data: x input; u input; xp output size=12; F1 input; Fneum1 input; F2 input; Fneum2 input; M1 input; M2 input; m parameter; Izz parameter; Jw parameter; Rg parameter; k_sus parameter; b_sus parameter; Iyy parameter; a1 parameter; a2 parameter; g parameter; h parameter
function xp  = G6_BiciDI_EE(x, u, F1, Fneum1, F2, Fneum2, M1, M2, m, Izz, Jw, Rg, k_sus, b_sus, Iyy, a1, a2, g, h)
% Modelo semi dinamico (o dinamico simple, ruedas con inercia)
% x: variables de estado [xcm_0, ycm_0, thetacm, vxcm, vycm, omegacm, wneum_1, wneum_2, psi, omegaycm, zcm, vzcm]'
% u: entradas [delta, Mu_1, Mu_2] --> delta es el angulo de direccion y
% Mu_1 Mu_2 son las torques de entrada sobre los neumaticos provistas
% por el motor/frenos
% F1(x,u) y F2(x,u): Fuerzas en los neumaticos delanteros y traseros. Son calculadas
% internamente al sistema por eso no van como entradas
% M1(x,u) y M2(x,u): Momentos sobre el CM producidos por los neumaticos
% xp: dx/dt = Ax + Bu + F(x,u)

cos_psi = cos(x(9));

A = [   0   0   0   cos(x(3))   -sin(x(3))  0   0   0   0   0   0   0
        0   0   0   sin(x(3))   cos(x(3))   0   0   0   0   0   0   0;
        0   0   0   0           0           1   0   0   0   0   0   0;
        0   0   0   0           0           0   0   0   0   0   0   0;
        0   0   0   0           0           0   0   0   0   0   0   0;
        0   0   0   0           0           0   0   0   0   0   0   0;
        0   0   0   0           0           0   0   0   0   0   0   0;
        0   0   0   0           0           0   0   0   0   0   0   0;
        0   0   0   0           0           0   0   0   0   1   0   0;
        0   0   0   0           0           0   0   0   0   -b_sus*(a1^2+a2^2)*cos_psi^2/Iyy   k_sus*(-a1+a2)*cos_psi/Iyy      b_sus*(-a1+a2)*cos_psi/Iyy;
        0   0   0   0           0           0   0   0   0   0   0   1;
        0   0   0   0           0           0   0   0   0   b_sus*(-a1+a2)*cos_psi/m   -2*k_sus/m    -2*b_sus/m;
        ];

B = [   0   0   0;
        0   0   0;
        0   0   0;
        0   0   0;
        0   0   0;
        0   0   0;
        0   1/Jw 0;
        0   0   1/Jw;
        0   0   0;
        0   0   0;
        0   0   0;
        0   0   0;
    ];

% Las fuerzas y momentos de los neumáticos los trabajo vectorialmente asi
% es mas facil agregar varias ruedas despues.
% Despues voy a pensar de hacer de esto algo como el 'calcVelOffset' porque
% la cuenta es la analoga.
Fres = F1 + F2; % Fuerza total. Se puede parametrizar fácil para varios neumaticos
Mres = M1 + M2; % Vector momento = suma de productos vectoriales

F = [   0;
    0;
    0;
    Fres(1)/m;
    Fres(2)/m;
    Mres(1)/Izz;
    -Fneum1(1)*Rg/Jw;
    -Fneum2(1)*Rg/Jw;
    0;
    (-k_sus*(a1^2 + a2^2)*cos_psi*sin(x(9)) + Fres(1) * (h+x(11))) / Iyy;
    0;
    -k_sus*(a1-a2)*sin(x(9))/m - g;
    ];

xp = A*x + B*u + F;

== matlab function ModG_Vehiculo/Bloque auto1/EE_G1 ==
  data: x input size=4; u input size=2; xp output size=4; L parameter size=1
function xp = G1_Bicicleta_EE(x,u, L)
% Ecuaciones de estado del cinemático puro de bicicleta
% x: vector de variables de estado [x2 y2 theta vx2]'
% u: vector de entradas            [ax2 delta]'
% xp: dx/dt = A(x,u)x + B(x)u
    A = [0  0   0   cos(x(3));
         0  0   0   sin(x(3));
         0  0   0   tan(u(2))/L;
         0  0   0   0];
     
    B = [0  0;
         0  0;
         0  0;
         1  0];
     
    xp = A*x + B*u;

== matlab function ModG_Vehiculo/Bloque auto1/ES_G1 ==
  data: x input size=4; y output; u input size=2
function y = G1_Bicicleta_ES(x, u)
% Ecuaciones de salida del cinemático puro de bicicleta
% x: vector de variables de estado [x2 y2 theta vx2]'
% y = Cx + Du
% y = [ v2x_0
%       v2y_0];
    C = [0  0   0   cos(x(3));      % v2x_0
         0  0   0   sin(x(3));];    % v2y_0
    D = [0  0;
         0  0;];

    y = C*x + D*u;

== matlab function ModG_Vehiculo/Bloque auto6/G6_BiciDI_ES ==
  data: x input; xy2 output size=2; v2_0 output size=2; a2 parameter size=1; a1 parameter; Fz1 output size=1; Fz2 output size=1; b_sus parameter; k_sus parameter
function [xy2, v2_0, Fz1, Fz2]  = G6_BiciDI_ES(x, a2, a1, b_sus, k_sus)
xy2 = [x(1) - a2*cos(x(3)); x(2) - a2*sin(x(3))];
v2_0 = [cos(x(3)) -sin(x(3)); sin(x(3)) cos(x(3))]*x(4:5);
Fz1 = k_sus* (-x(11) - a1 * sin(x(9))) - b_sus *(-x(12) - a1 * x(10) * cos(x(9)));
Fz2 = k_sus* (-x(11) + a2 * sin(x(9))) - b_sus *(-x(12) + a2 * x(10) * cos(x(9)));

== matlab function ModG_Vehiculo/Bloque auto 7 /G7_Ultimo_EE ==
  data m settings: description=Masa del auto
  data Izz settings: description=Momento de inercia en el eje z respecto al cm
  data: x input; u input; xp output size=10; Fneums input; Fneums_cm input; Mneums_cm input; m parameter; Izz parameter; Jw parameter; Rg parameter; a1 parameter; a2 parameter; b_sus parameter; k_sus parameter; Iyy parameter
function xp  = G7_Ultimo_EE(x, u, Fneums, Fneums_cm, Mneums_cm, m, Izz, Jw, Rg, a1, a2, b_sus, k_sus, Iyy)
% Modelo 4 ruedas dinamicas
% x: variables de estado
%[xcm_0, ycm_0, thetacm, vxcm, vycm, omegacm, wneum_1d, wneum_1i, wneum_2d, wneum_2i]'
%[  1      2       3      4     5       6       7           8       9   10]
% u: entradas [delta, Mu_1, Mu_2] --> delta es el angulo de direccion y
% Mu_1 Mu_2 son las torques de entrada sobre los ejes delanteros y traseros
% provistas por el motor
% Fneums: Fuerzas en los neumaticos vistas en su propio sistema
% Fneums_cm: Fuerzas en los neumaticos vistas del sistema CM
% Mneums_cm: Momentos producidos por los neumáticos sobre el CM
% xp: dx/dt = Ax + Bu + F(x,u)

cos_psi = cos(x(11));

A = [   0   0   0   cos(x(3))   -sin(x(3))  0   0   0   0   0   0   0   0   0;
        0   0   0   sin(x(3))   cos(x(3))   0   0   0   0   0   0   0   0   0;
        0   0   0   0           0           1   0   0   0   0   0   0   0   0;
        0   0   0   0           0           0   0   0   0   0   0   0   0   0;
        0   0   0   0           0           0   0   0   0   0   0   0   0   0;
        0   0   0   0           0           0   0   0   0   0   0   0   0   0;
        0   0   0   0           0           0   0   0   0   0   0   0   0   0;
        0   0   0   0           0           0   0   0   0   0   0   0   0   0;
        0   0   0   0           0           0   0   0   0   0   0   0   0   0;
        0   0   0   0           0           0   0   0   0   0   0   0   0   0;
        0   0   0   0           0           0   0   0   0   0   0   1   0   0;
        0   0   0   0           0           0   0   0   0   0   0   -b_sus*(a1^2+a2^2)*cos_psi^2/Iyy   k_sus*(-a1+a2)*cos_psi/Iyy      b_sus*(-a1+a2)*cos_psi/Iyy;
        0   0   0   0           0           0   0   0   0   0   0   0   0   1;
        0   0   0   0           0           0   0   0   0   0   0   b_sus*(-a1+a2)*cos_psi/m   -2*k_sus/m    -2*b_sus/m;
    ];

B = [   0   0   0;
    0   0   0;
    0   0   0;
    0   0   0;
    0   0   0;
    0   0   0;
    0   1/Jw 0;
    0   1/Jw 0;
    0   0   1/Jw;
    0   0   1/Jw;
    ];

% Las fuerzas de neumaticos vienen en matrices de 3xn donde cada columna
% representa el vector fuerza (o momento o velocidad cuando corresponda)
% del neumatico. El orden de estos vectores de la forma:
% Fneums = [F1d, F1i, F2d, F2i] = [Del-Der, Del-Izq, Tra-Der, Tra-Izq]
Fneums = reshape(Fneums, 3,4);
Fneums_cm = reshape(Fneums_cm, 2,4);
%Mneums_cm = reshape(Mneums_cm, 3,4);
Fres = sum(Fneums_cm'); % Fuerza total sobre el CM producida por los neumaticos
Mres = sum(Mneums_cm'); % Momento total sobre el CM producido por los neumaticos

F = [   0;
    0;
    0;
    Fres(1)/m;
    Fres(2)/m;
    Mres(1)/Izz;
    -Fneums(1,1)*Rg/Jw;
    -Fneums(1,2)*Rg/Jw;
    -Fneums(1,3)*Rg/Jw;
    -Fneums(1,4)*Rg/Jw;
    0;
    -k_sus*(a1^2 + a2^2)*cos_psi*sin(x(11)) + Fres(1) * (h+x(11)) / Iyy;
    0;
    -k_sus*(a1-a2)*sin(x(11))/m - g;
    ];
    
xp = A*x + B*u + F;

== matlab function ModG_Vehiculo/Bloque auto 7 /G7_Ultimo_ES ==
  data: x input; phix input; phiy input; vpunto input; xy2 output size=2; v2_0 output size=2; a2 parameter size=1; Fz1234 output; a1 parameter; m parameter; g parameter; h parameter; L parameter; b1d parameter; b1i parameter; b2d parameter; b2i parameter; T1 parameter; T2 parameter; k_sus parameter; b_sus parameter
function [xy2, v2_0, Fz1234]  = G7_Ultimo_ES(x, phix, phiy, vpunto, a2, a1, m, g, h, L, b1d, b1i, b2d, b2i, T1, T2, k_sus, b_sus)
xy2 = [x(1) - a2*cos(x(3)); x(2) - a2*sin(x(3))];
v2_0 = [cos(x(3)) -sin(x(3)); sin(x(3)) cos(x(3))]*x(4:5);
%Fz1 = m*g*(a2/L * cos(phix) - h/L * sin(phix)); % Estas 2 lineas son sin termino de aceleracion para evitar lazo algebraico
%Fz2 = m*g*(a1/L * cos(phix) + h/L * sin(phix)); % Estas 2 lineas son sin termino de aceleracion para evitar lazo algebraico
%El modelo del auto no es 3d, si no que son 3 submodelos 2d. 1 modelo
%longitudinal y 2 modelos laterales en cada eje. Entonces primero se
%calcula la fuerza normal sobre el eje delantero y trasero con el modelo
%longitudinal y luego esa Fz representa el peso del auto para el calculo de
%transferencia de peso lateral
Fz1 = k_sus* (-x(13) - a1 * sin(x(11))) - b_sus *(-x(14) - a1 * x(12) * cos(x(11)));
Fz2 = k_sus* (-x(13) + a2 * sin(x(11))) - b_sus *(-x(14) + a2 * x(12) * cos(x(11)));
Fz1d = Fz1*(b1i/T1 * cos(phiy) + h/T1 * sin(phiy)) + Fz1/g*vpunto(2)*h/T1;
Fz1i = Fz1*(b1d/T1 * cos(phiy) - h/T1 * sin(phiy)) - Fz1/g*vpunto(2)*h/T1;
Fz2d = Fz2*(b2i/T2 * cos(phiy) + h/T2 * sin(phiy)) + Fz2/g*vpunto(2)*h/T2;
Fz2i = Fz2*(b2d/T2 * cos(phiy) - h/T2 * sin(phiy)) - Fz2/g*vpunto(2)*h/T2;
Fz1234 = [Fz1d, Fz1i, Fz2d, Fz2i]';
